simulink model "MultiRobotPaintingModel_fixed"  (R2025b)
settings: Solver=ode23t  StartTime=0.0  StopTime=inf  MaxStep=0.01  RelTol=1e-3
InitFcn:
  | init_MultiRobotPaintingModel
model workspace (MAT data in the model file):
  OPCUA_ENDPOINT = 'opc.tcp://localhost:4840'
  OPCUA_NS = 2
undefined symbols (not defined in the file): Kp_joint, PLC_1, SIMATIC, UA
libraries: opcualib x2
settings Model: Creator=SYNAPTICON  LastModifiedBy=Almat
settings DataIOCC: SaveOutput=off
settings DebuggingCC: UnderspecifiedInitializationDetection=Classic  MergeDetectMultiDrivingBlocksExec=none
settings ModelReferenceCC: PropagateSignalLabelsOutOfModel=off

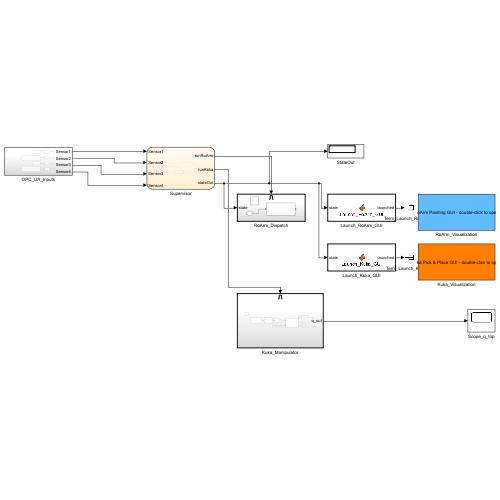
[thumbnail: Simulink's stored preview of the top-level diagram]
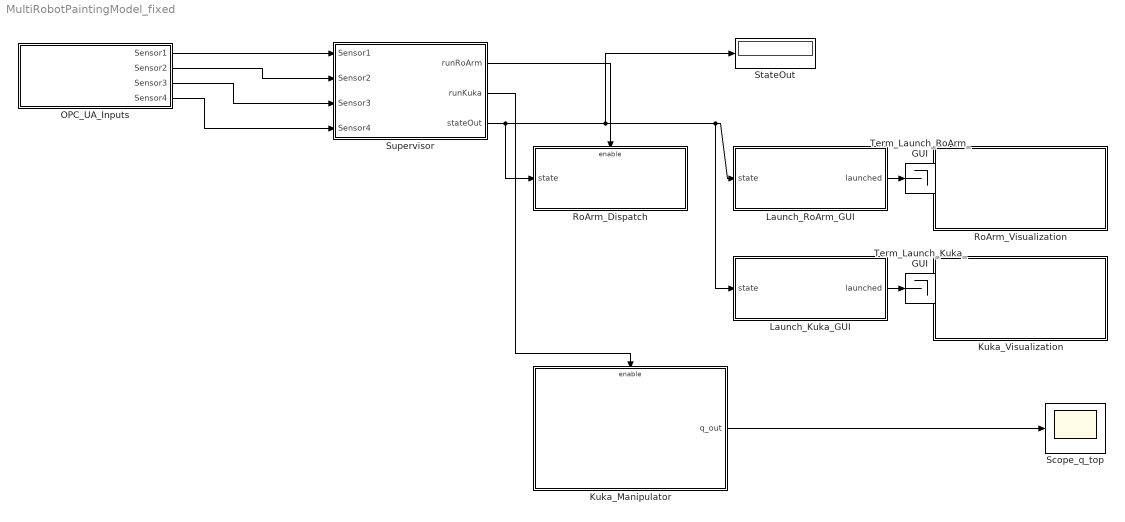
== system MultiRobotPaintingModel_fixed ==
  Kuka_Manipulator : Subsystem
  Kuka_Visualization : Subsystem  mask(Kuka_Visualization){}
      mask help:
      | Kuka_Visualization
      |
      | Double-click this block to open the GUI manually,
      | or trigger the corresponding sensor on the PLC to have
      | Simulink open it automatically.
      settings: OpenFcn=kuka_pick_and_place_gui;
      mask Display:
      | color('black')
      | disp('Kuka Pick & Place GUI - double-click to open')
  Launch_Kuka_GUI : MATLAB Function  TreatAsAtomicUnit=on
  Launch_RoArm_GUI : MATLAB Function  TreatAsAtomicUnit=on
  OPC_UA_Inputs : Subsystem
  RoArm_Dispatch : Subsystem
  RoArm_Visualization : Subsystem  mask(RoArm_Visualization){}
      mask help:
      | RoArm_Visualization
      |
      | Double-click this block to open the GUI manually,
      | or trigger the corresponding sensor on the PLC to have
      | Simulink open it automatically.
      settings: OpenFcn=roarms_painting_process_gui;
      mask Display:
      | color('black')
      | disp('RoArm Painting GUI - double-click to open')
  Scope_q_top : Scope
  StateOut : Display
  Supervisor : Stateflow chart  TreatAsAtomicUnit=on
  Term_Launch_Kuka_GUI : Terminator
  Term_Launch_RoArm_GUI : Terminator
  wires:
  OPC_UA_Inputs/1(Sensor1) -> Supervisor/1(Sensor1)
  OPC_UA_Inputs/2(Sensor2) -> Supervisor/2(Sensor2)
  OPC_UA_Inputs/3(Sensor3) -> Supervisor/3(Sensor3)
  OPC_UA_Inputs/4(Sensor4) -> Supervisor/4(Sensor4)
  Supervisor/1(runRoArm) -> RoArm_Dispatch/Enable
  Supervisor/3(stateOut) -> Launch_RoArm_GUI/1(state), Launch_Kuka_GUI/1(state), StateOut/1, RoArm_Dispatch/1(state)
  Supervisor/2(runKuka) -> Kuka_Manipulator/Enable
  Launch_RoArm_GUI/1(launched) -> Term_Launch_RoArm_GUI/1
  Launch_Kuka_GUI/1(launched) -> Term_Launch_Kuka_GUI/1
  Kuka_Manipulator/1(q_out) -> Scope_q_top/1

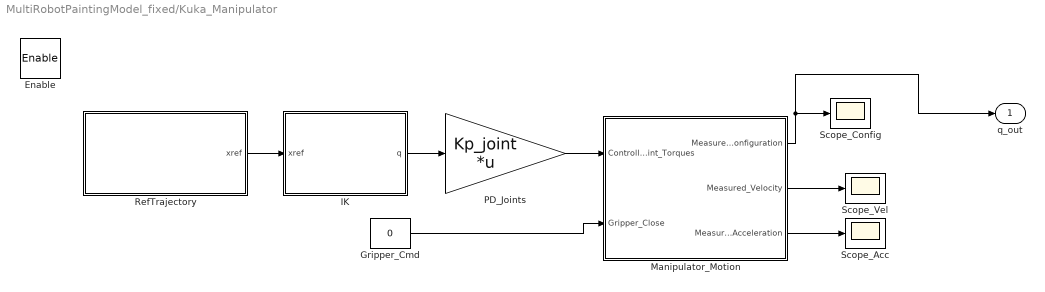
== system MultiRobotPaintingModel_fixed/Kuka_Manipulator ==
  Enable : EnablePort
  Gripper_Cmd : Constant  Value=0
  IK : MATLAB Function  TreatAsAtomicUnit=on
  Manipulator_Motion : Subsystem
  PD_Joints : Gain  Gain=Kp_joint  Multiplication=Matrix(K*u)
  RefTrajectory : MATLAB Function  TreatAsAtomicUnit=on
  Scope_Acc : Scope
  Scope_Config : Scope
  Scope_Vel : Scope
  q_out : Outport
  wires:
  Gripper_Cmd/1 -> Manipulator_Motion/2(Gripper_Close)
  RefTrajectory/1(xref) -> IK/1(xref)
  IK/1(q) -> PD_Joints/1
  PD_Joints/1 -> Manipulator_Motion/1(Controller_Joint_Torques)
  Manipulator_Motion/1(Measured_Configuration) -> Scope_Config/1, q_out/1
  Manipulator_Motion/2(Measured_Velocity) -> Scope_Vel/1
  Manipulator_Motion/3(Measured_Acceleration) -> Scope_Acc/1

== system MultiRobotPaintingModel_fixed/Kuka_Visualization ==

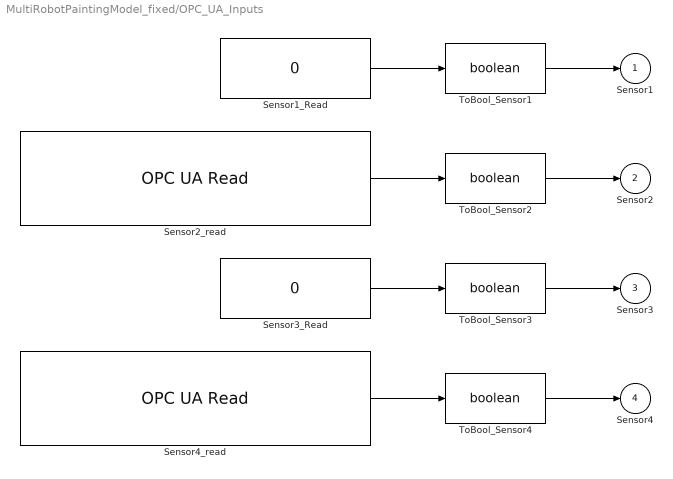
== system MultiRobotPaintingModel_fixed/OPC_UA_Inputs ==
  Sensor1_Read : Constant  Value=0  OutDataTypeStr=boolean
  Sensor2_read : opcualib/OPC UA Read  SelectedServer=SIMATIC.S7-1500.OPC-UA.Application:PLC_1  ServerList=SIMATIC.S7-1500.OPC-UA.Application:PLC_1  NodeList={ '1', 'Read_value1_to_Matlab', '4', '2', '1' }  ShowQualityPort=off  ShowTimestampPort=off  ShowTimestampPortAs=Seconds since start  SampleTime=10
  Sensor3_Read : Constant  Value=0  OutDataTypeStr=boolean
  Sensor4_read : opcualib/OPC UA Read  SelectedServer=SIMATIC.S7-1500.OPC-UA.Application:PLC_1  ServerList=SIMATIC.S7-1500.OPC-UA.Application:PLC_1  NodeList={ '1', 'Read_value2_to_Matlab', '4', '3', '1' }  ShowQualityPort=off  ShowTimestampPort=off  ShowTimestampPortAs=Seconds since start  SampleTime=10
  ToBool_Sensor{1..4} (4 alike) : DataTypeConversion  OutDataTypeStr=boolean  SaturateOnIntegerOverflow=off  RndMeth=Floor
  Sensor1 : Outport  OutDataTypeStr=boolean
  Sensor2 : Outport  Port=2  OutDataTypeStr=boolean
  Sensor3 : Outport  Port=3  OutDataTypeStr=boolean
  Sensor4 : Outport  Port=4  OutDataTypeStr=boolean
  wires:
  Sensor1_Read/1 -> ToBool_Sensor1/1
  ToBool_Sensor1/1 -> Sensor1/1
  Sensor2_read/1 -> ToBool_Sensor2/1
  ToBool_Sensor2/1 -> Sensor2/1
  Sensor3_Read/1 -> ToBool_Sensor3/1
  ToBool_Sensor3/1 -> Sensor3/1
  Sensor4_read/1 -> ToBool_Sensor4/1
  ToBool_Sensor4/1 -> Sensor4/1

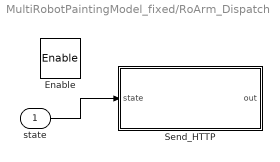
== system MultiRobotPaintingModel_fixed/RoArm_Dispatch ==
  state : Inport
  Enable : EnablePort
  Send_HTTP : MATLAB Function  TreatAsAtomicUnit=on
  wires:
  state/1 -> Send_HTTP/1(state)

== system MultiRobotPaintingModel_fixed/RoArm_Visualization ==

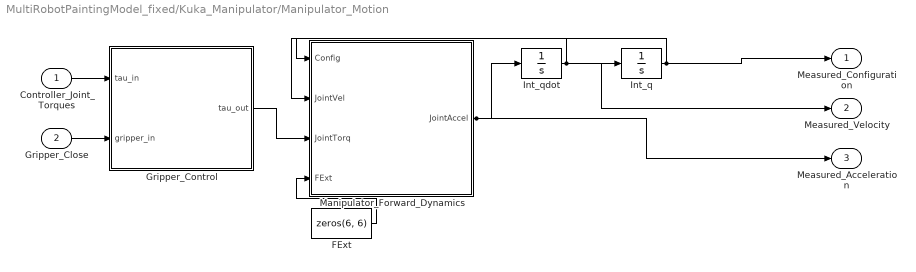
== system MultiRobotPaintingModel_fixed/Kuka_Manipulator/Manipulator_Motion ==
  Controller_Joint_Torques : Inport
  Gripper_Close : Inport  Port=2
  FExt : Constant  Value=zeros(6, 6)  OutDataTypeStr=double
  Gripper_Control : Subsystem
  Int_q : Integrator  InitialCondition=zeros(6,1)
  Int_qdot : Integrator  InitialCondition=zeros(6,1)
  Manipulator_Forward_Dynamics : MATLAB Function  TreatAsAtomicUnit=on
  Measured_Configuration : Outport
  Measured_Velocity : Outport  Port=2
  Measured_Acceleration : Outport  Port=3
  wires:
  Controller_Joint_Torques/1 -> Gripper_Control/1(tau_in)
  Gripper_Close/1 -> Gripper_Control/2(gripper_in)
  Gripper_Control/1(tau_out) -> Manipulator_Forward_Dynamics/3(JointTorq)
  Int_q/1 -> Manipulator_Forward_Dynamics/1(Config), Measured_Configuration/1
  Int_qdot/1 -> Manipulator_Forward_Dynamics/2(JointVel), Int_q/1, Measured_Velocity/1
  FExt/1 -> Manipulator_Forward_Dynamics/4(FExt)
  Manipulator_Forward_Dynamics/1(JointAccel) -> Int_qdot/1, Measured_Acceleration/1

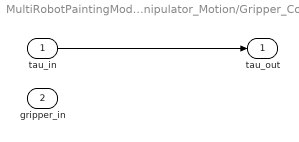
== system MultiRobotPaintingModel_fixed/Kuka_Manipulator/Manipulator_Motion/Gripper_Control ==
  tau_in : Inport
  gripper_in : Inport  Port=2
  tau_out : Outport
  wires:
  tau_in/1 -> tau_out/1

== matlab function MultiRobotPaintingModel_fixed/Kuka_Manipulator/RefTrajectory ==
  data: xref output
function xref = RefTrajectory()
%#codegen
persistent t0
if isempty(t0), t0 = 0; end
t0 = t0 + 0.01;
cx = 0.60; cy = 0.10; cz = 0.40; r = 0.12;
xref = [cx + r*cos(t0); cy + r*sin(t0); cz; 0; pi/2; 0];
end

== matlab function MultiRobotPaintingModel_fixed/RoArm_Dispatch/Send_HTTP ==
  data: state input; out output
function out = Send_HTTP(state)
%#codegen
coder.extrinsic('webwrite','weboptions');
out = uint8(state);
if coder.target('MATLAB')
    opts = weboptions('Timeout', 2, 'MediaType','application/json');
    % Move RoArm to a painting-ready pose each time the dispatcher is enabled
    webwrite('http://192.168.0.192/js', ...
             '{"T":1041,"x":250,"y":0,"z":150,"t":3.14,"r":0}', opts);
end
end

== stateflow chart MultiRobotPaintingModel_fixed/Supervisor ==
  state KUKA_ACTIVE
    entry: runRoArm = false; runKuka = true; stateOut = uint8(2);
  state IDLE
    entry: runRoArm = false; runKuka = false; stateOut = uint8(0);
  state ROARM_ACTIVE
    entry: runRoArm = true; runKuka = false; stateOut = uint8(1);
  KUKA_ACTIVE -> IDLE : [Sensor4 == false && Sensor2 == false]
  ROARM_ACTIVE -> IDLE [order 2] : [Sensor2 == false]
  (default) -> IDLE
  ROARM_ACTIVE -> KUKA_ACTIVE [order 1] : [Sensor4 == true]
  IDLE -> ROARM_ACTIVE : [Sensor2 == true]
  data: Sensor1 input boolean; Sensor2 input boolean; Sensor3 input boolean; Sensor4 input boolean; runRoArm output boolean; runKuka output boolean; stateOut output uint8

== matlab function MultiRobotPaintingModel_fixed/Kuka_Manipulator/IK ==
  data: xref input; q output
function q = IK(xref)
%#codegen
% Simple analytic surrogate: project the Cartesian reference into
% joint angles via per-axis gains so downstream blocks see a
% non-zero, smooth signal even without the IK block.
K = [1.5; 1.2; 1.0; 0.8; 0.6; 0.4];
q = K .* xref;
end

== matlab function MultiRobotPaintingModel_fixed/Kuka_Manipulator/Manipulator_Motion/Manipulator_Forward_Dynamics ==
  data: Config input; JointAccel output; JointVel input; JointTorq input; FExt input
function JointAccel = Manipulator_Forward_Dynamics(Config, JointVel, JointTorq, FExt) %#ok<INUSD>
%#codegen
M = diag([4 5 4 2 1.5 1]);    % lumped joint inertia
D = diag([2 2 2 1 1 0.5]);    % viscous damping
G = 0.05 * [sin(Config(2)); cos(Config(3)); 0; 0; 0; 0];  % mock gravity term
JointAccel = M \ (JointTorq - D*JointVel - G);
end

== matlab function MultiRobotPaintingModel_fixed/Launch_RoArm_GUI ==
  data: state input; launched output
function launched = Launch_RoArm_GUI(state)
%#codegen
coder.extrinsic('evalin','disp','drawnow');

persistent prev

if isempty(prev)
    prev = uint8(0);
end

state = uint8(state);
launched = false;

if state == uint8(1) && prev ~= uint8(1)
    disp('[Simulink] Launching RoArm GUI...');
    evalin('base', ...
        ['addpath(''C:\Users\Almat\Documents\MATLAB\MATLAB_updated\MATLAB\MultiRobot\MultiRobot'',''-begin''); ' ...
        'rehash; ' ...
        'roarms_painting_process(true);']);
    drawnow;
    launched = true;
end

prev = state;
end

== matlab function MultiRobotPaintingModel_fixed/Launch_Kuka_GUI ==
  data: state input; launched output
function launched = Launch_Kuka_GUI(state)
%#codegen
coder.extrinsic('evalin','disp','drawnow');

persistent prev

if isempty(prev)
    prev = uint8(0);
end

state = uint8(state);
launched = false;

if state == uint8(2) && prev ~= uint8(2)
    disp('[Simulink] Launching KUKA GUI...');
    evalin('base', ...
        ['addpath(''C:\Users\Almat\Documents\MATLAB\MATLAB_updated\MATLAB\MultiRobot\MultiRobot'',''-begin''); ' ...
        'rehash; ' ...
        'kuka_pick_and_place_gui_magnetic(true);']);
    drawnow;
    launched = true;
end

prev = state;
end
